simulink model "pathNavigation_PID_VEX"  (R2017a)
settings: Solver=FixedStepAuto  StartTime=0.0  StopTime=inf  FixedStep=Ts  RelTol=1e-3  EnableMultiTasking=on
PreLoadFcn:
  | robotParameters;
undefined symbols (not defined in the file or in its folder): axleLength, motorIp, motorSp, ticksPerRot, Ts, wheelR
libraries: vexarmcortexlib x8, simulink x2, simulink_extras x1, mobileRoboticsTrainingLib x1
settings Model: ExtModeTrigDuration=25  Creator=sseshadr  LastModifiedBy=shiremat
settings OptimizationCC: PassReuseOutputArgsAs=Individual arguments  MaxStackSize=64
settings DebuggingCC: ParameterTunabilityLossMsg=error
settings HardwareCC: ProdBitPerPointer=32  ProdBitPerSizeT=32  ProdBitPerPtrDiffT=32  ProdLargestAtomicInteger=Long  ProdLargestAtomicFloat=Double  ProdWordSize=32  ProdHWDeviceType=ARM Compatible->ARM Cortex
settings SFSimCC: MATLABDynamicMemAlloc=off
settings RTWCC: SystemTargetFile=ert.tlc  HardwareBoard=ARM Cortex-based VEX Microcontroller  TLCOptions="-aInlineSetEventsForThisBaseRateFcn=TLC_FALSE -aSuppressMultiTaskScheduler=TLC_FALSE  -aRateBasedStepFcn=0"  TemplateMakefile=ert_default_tmf  Description=Embedded Coder  GenerateReport=on  Toolchain=GNU Tools for VEX ARM Cortex  IncludeHyperlinkInReport=on  LaunchReport=on  GenerateTraceInfo=on  GenerateTraceReport=on  GenerateTraceReportSl=on  GenerateTraceReportSf=on  GenerateTraceReportEml=on
settings CodeAppCC: ForceParamTrailComments=on  IgnoreCustomStorageClasses=off  OperatorAnnotations=on  SimulinkDataObjDesc=on  SFDataObjDesc=on  MATLABFcnDesc=on  InsertBlockDesc=on  MATLABSourceComments=on

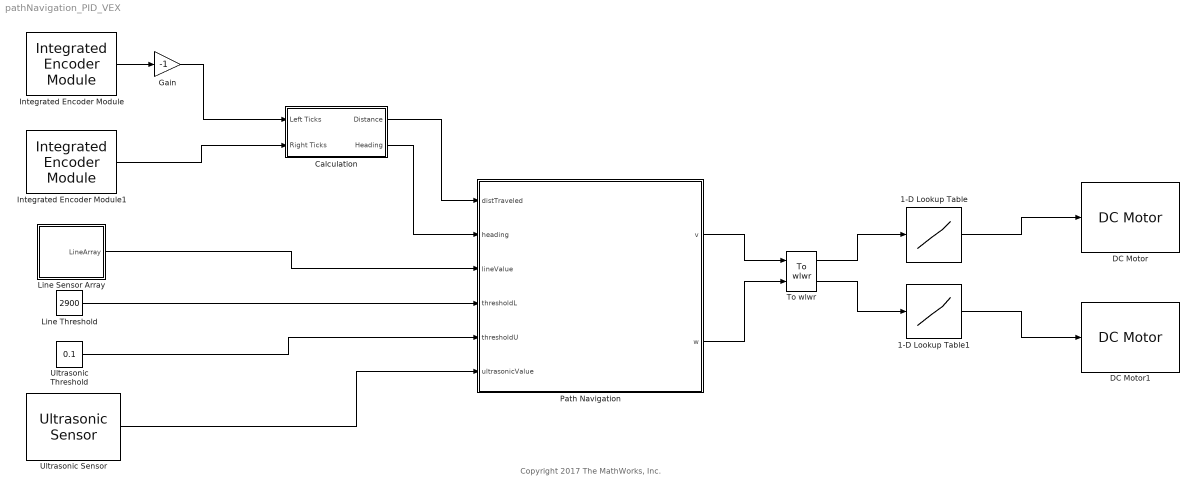
== system pathNavigation_PID_VEX ==
  note: Copyright 2017 The MathWorks, Inc.
  1-D Lookup Table : Lookup_n-D  NumberOfTableDimensions=1  BreakpointsForDimension1=motorSp  Table=motorIp  ExtrapMethod=Clip  InternalRulePriority=Speed  RndMeth=Simplest  InputSameDT=on
  1-D Lookup Table1 : Lookup_n-D  NumberOfTableDimensions=1  BreakpointsForDimension1=motorSp  Table=motorIp  ExtrapMethod=Clip  InternalRulePriority=Speed  RndMeth=Simplest  InputSameDT=on
  Calculation : Subsystem
  DC Motor : vexarmcortexlib/Actuators/DC Motor  motor=10  scaleFactor=1/13.5  SimulationOut=off
      settings: SourceProductName=Simulink Coder Support Package for ARM Cortex-based VEX Microcontroller  SourceProductBaseCode=EC_VEX_MICRO
  DC Motor1 : vexarmcortexlib/Actuators/DC Motor  motor=1  scaleFactor=1/13.5  SimulationOut=off
      settings: SourceProductName=Simulink Coder Support Package for ARM Cortex-based VEX Microcontroller  SourceProductBaseCode=EC_VEX_MICRO
  Gain : Gain  Gain=-1
  Integrated Encoder Module : vexarmcortexlib/Sensors/Integrated Encoder Module  motorType=VEX 393 (High torque)  seqNumI2C=1  resetOption=No reset  rotVelocity=off  inputPortSim=off  SampleTime=Ts
      settings: SourceProductName=Simulink Coder Support Package for ARM Cortex-based VEX Microcontroller  SourceProductBaseCode=EC_VEX_MICRO
  Integrated Encoder Module1 : vexarmcortexlib/Sensors/Integrated Encoder Module  motorType=VEX 393 (High torque)  seqNumI2C=0  resetOption=No reset  rotVelocity=off  inputPortSim=off  SampleTime=Ts
      settings: SourceProductName=Simulink Coder Support Package for ARM Cortex-based VEX Microcontroller  SourceProductBaseCode=EC_VEX_MICRO
  Line Sensor Array : Subsystem
  Line Threshold : Constant  Value=2900
  Path Navigation : Stateflow chart  TreatAsAtomicUnit=on
  To wlwr : mobileRoboticsTrainingLib/To wlwr  axleLength=axleLength  wheelR=wheelR
  Ultrasonic Sensor : vexarmcortexlib/Sensors/Ultrasonic Sensor  inputPin=7  outputPin=6  inputPortSim=off  SampleTime=Ts
      settings: SourceProductName=Simulink Coder Support Package for ARM Cortex-based VEX Microcontroller  SourceProductBaseCode=EC_VEX_MICRO
  Ultrasonic Threshold : Constant  Value=0.1
  wires:
  1-D Lookup Table1/1 -> DC Motor1/1
  1-D Lookup Table/1 -> DC Motor/1
  To wlwr/1 -> 1-D Lookup Table/1
  To wlwr/2 -> 1-D Lookup Table1/1
  Path Navigation/1(v) -> To wlwr/1
  Path Navigation/2(w) -> To wlwr/2
  Ultrasonic Sensor/1 -> Path Navigation/6(ultrasonicValue)
  Integrated Encoder Module1/1 -> Calculation/2(Right Ticks)
  Integrated Encoder Module/1 -> Gain/1
  Calculation/1(Distance) -> Path Navigation/1(distTraveled)
  Calculation/2(Heading) -> Path Navigation/2(heading)
  Line Threshold/1 -> Path Navigation/4(thresholdL)
  Ultrasonic Threshold/1 -> Path Navigation/5(thresholdU)
  Gain/1 -> Calculation/1(Left Ticks)
  Line Sensor Array/1(LineArray) -> Path Navigation/3(lineValue)

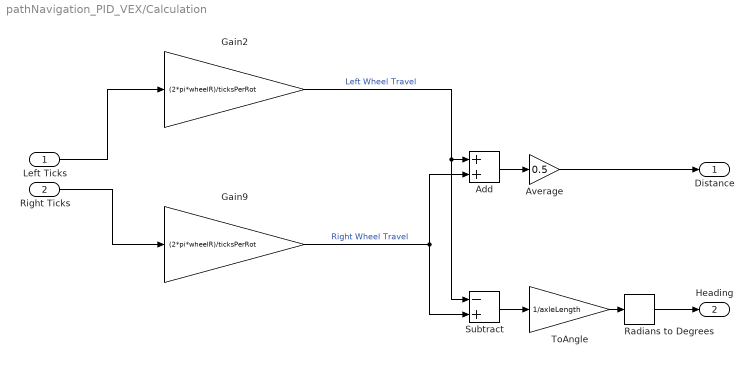
== system pathNavigation_PID_VEX/Calculation ==
  Left Ticks : Inport
  Right Ticks : Inport  Port=2
  Add : Sum
  Average : Gain  Gain=0.5
  Gain2 : Gain  Gain=(2*pi*wheelR)/ticksPerRot
  Gain9 : Gain  Gain=(2*pi*wheelR)/ticksPerRot
  Radians to Degrees : simulink_extras/Transformations/Radians to Degrees
  Subtract : Sum  Inputs=-+
  ToAngle : Gain  Gain=1/axleLength
  Distance : Outport
  Heading : Outport  Port=2
  wires:
  Average/1 -> Distance/1
  Add/1 -> Average/1
  Gain2/1 -> Subtract/1, Add/1  "Left Wheel Travel"
  Right Ticks/1 -> Gain9/1
  Left Ticks/1 -> Gain2/1
  Gain9/1 -> Subtract/2, Add/2  "Right Wheel Travel"
  Subtract/1 -> ToAngle/1
  ToAngle/1 -> Radians to Degrees/1
  Radians to Degrees/1 -> Heading/1

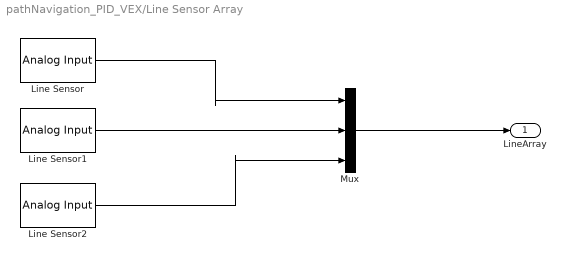
== system pathNavigation_PID_VEX/Line Sensor Array ==
  Line Sensor : vexarmcortexlib/Sensors/Analog Input  inChan=8  SimulationIn=off  SampleTime=Ts
      settings: SourceProductName=Simulink Coder Support Package for ARM Cortex-based VEX Microcontroller  SourceProductBaseCode=EC_VEX_MICRO
  Line Sensor1 : vexarmcortexlib/Sensors/Analog Input  inChan=7  SimulationIn=off  SampleTime=Ts
      settings: SourceProductName=Simulink Coder Support Package for ARM Cortex-based VEX Microcontroller  SourceProductBaseCode=EC_VEX_MICRO
  Line Sensor2 : vexarmcortexlib/Sensors/Analog Input  inChan=6  SimulationIn=off  SampleTime=Ts
      settings: SourceProductName=Simulink Coder Support Package for ARM Cortex-based VEX Microcontroller  SourceProductBaseCode=EC_VEX_MICRO
  Mux : Mux  Inputs=3
  LineArray : Outport
  wires:
  Line Sensor1/1 -> Mux/2
  Line Sensor/1 -> Mux/1
  Line Sensor2/1 -> Mux/3
  Mux/1 -> LineArray/1

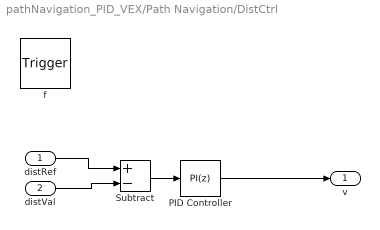
== system pathNavigation_PID_VEX/Path Navigation/DistCtrl ==
  distRef : Inport  OutDataTypeStr=double  PortDimensions=1
  distVal : Inport  Port=2  OutDataTypeStr=double  PortDimensions=1
  f : TriggerPort  TriggerType=function-call  VariantControl=Variant
      settings: CopyFcn=Stateflow.SLINSF.SimulinkMan.removeBlockPreDeleteFcn  PreDeleteFcn=Stateflow.SLINSF.SimulinkMan.unsafePredeleteFcn
  PID Controller : simulink/Continuous/PID Controller  Controller=PI  TimeDomain=Discrete-time  SampleTime=-1  IntegratorMethod=Forward Euler  FilterMethod=Forward Euler  Form=Parallel  UseFilter=off  ControllerParametersSource=internal  P=1.1  I=0.2  D=-0.0140783779685636  N=151.701833251505  InitialConditionSource=internal  InitialConditionForIntegrator=0  InitialConditionForFilter=0  ExternalReset=none  LimitOutput=on  UpperSaturationLimit=0.6  LowerSaturationLimit=-0.6  LinearizeAsGain=on  AntiWindupMode=clamping  Kb=1  TrackingMode=off  Kt=1  PParamMin=[]  PParamMax=[]  IParamMin=[]  IParamMax=[]  DParamMin=[]  DParamMax=[]  NParamMin=[]  NParamMax=[]  KbParamMin=[]  KbParamMax=[]  KtParamMin=[]  KtParamMax=[]  POutMin=[]  POutMax=[]  IOutMin=[]  IOutMax=[]  DOutMin=[]  DOutMax=[]  NOutMin=[]  NOutMax=[]  KbOutMin=[]  KbOutMax=[]  KtOutMin=[]  KtOutMax=[]  IntegratorOutMin=[]  IntegratorOutMax=[]  FilterOutMin=[]  FilterOutMax=[]  SumOutMin=[]  SumOutMax=[]  SumI1OutMin=[]  SumI1OutMax=[]  SumI2OutMin=[]  SumI2OutMax=[]  SumI3OutMin=[]  SumI3OutMax=[]  SumDOutMin=[]  SumDOutMax=[]  SaturationOutMin=[]  SaturationOutMax=[]  IntegratorContinuousStateAttributes=''  IntegratorStateMustResolveToSignalObject=off  IntegratorRTWStateStorageClass=Auto  FilterContinuousStateAttributes=''  FilterStateMustResolveToSignalObject=off  FilterRTWStateStorageClass=Auto  DifferentiatorICPrevScaledInput=0  DifferentiatorOutMin=[]  DifferentiatorOutMax=[]  InitialConditionSetting=Output
  Subtract : Sum  Inputs=+-
  v : Outport
  wires:
  Subtract/1 -> PID Controller/1
  PID Controller/1 -> v/1
  distRef/1 -> Subtract/1
  distVal/1 -> Subtract/2

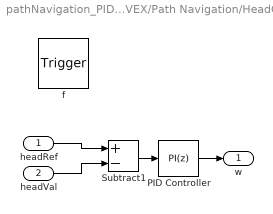
== system pathNavigation_PID_VEX/Path Navigation/HeadCtrl ==
  headRef : Inport  OutDataTypeStr=double  PortDimensions=1
  headVal : Inport  Port=2  OutDataTypeStr=double  PortDimensions=1
  f : TriggerPort  TriggerType=function-call  VariantControl=Variant
      settings: CopyFcn=Stateflow.SLINSF.SimulinkMan.removeBlockPreDeleteFcn  PreDeleteFcn=Stateflow.SLINSF.SimulinkMan.unsafePredeleteFcn
  PID Controller : simulink/Continuous/PID Controller  Controller=PI  TimeDomain=Discrete-time  SampleTime=-1  IntegratorMethod=Forward Euler  FilterMethod=Forward Euler  Form=Parallel  UseFilter=off  ControllerParametersSource=internal  P=0.1  I=0.1  D=-0.0140783779685636  N=151.701833251505  InitialConditionSource=internal  InitialConditionForIntegrator=0  InitialConditionForFilter=0  ExternalReset=none  LimitOutput=on  UpperSaturationLimit=4  LowerSaturationLimit=-4  LinearizeAsGain=on  AntiWindupMode=clamping  Kb=1  TrackingMode=off  Kt=1  PParamMin=[]  PParamMax=[]  IParamMin=[]  IParamMax=[]  DParamMin=[]  DParamMax=[]  NParamMin=[]  NParamMax=[]  KbParamMin=[]  KbParamMax=[]  KtParamMin=[]  KtParamMax=[]  POutMin=[]  POutMax=[]  IOutMin=[]  IOutMax=[]  DOutMin=[]  DOutMax=[]  NOutMin=[]  NOutMax=[]  KbOutMin=[]  KbOutMax=[]  KtOutMin=[]  KtOutMax=[]  IntegratorOutMin=[]  IntegratorOutMax=[]  FilterOutMin=[]  FilterOutMax=[]  SumOutMin=[]  SumOutMax=[]  SumI1OutMin=[]  SumI1OutMax=[]  SumI2OutMin=[]  SumI2OutMax=[]  SumI3OutMin=[]  SumI3OutMax=[]  SumDOutMin=[]  SumDOutMax=[]  SaturationOutMin=[]  SaturationOutMax=[]  IntegratorContinuousStateAttributes=''  IntegratorStateMustResolveToSignalObject=off  IntegratorRTWStateStorageClass=Auto  FilterContinuousStateAttributes=''  FilterStateMustResolveToSignalObject=off  FilterRTWStateStorageClass=Auto  DifferentiatorICPrevScaledInput=0  DifferentiatorOutMin=[]  DifferentiatorOutMax=[]  InitialConditionSetting=Output
  Subtract1 : Sum  Inputs=+-
  w : Outport
  wires:
  Subtract1/1 -> PID Controller/1
  PID Controller/1 -> w/1
  headRef/1 -> Subtract1/1
  headVal/1 -> Subtract1/2

== stateflow chart pathNavigation_PID_VEX/Path Navigation ==
  state SegmentA
    state MoveForward
      entry:
      v = DistCtrl(1.05,distTraveled);
    state Stop
      entry:
      v = 0;
    state Rotate
      entry:
      w = HeadCtrl(-85,heading);
    state Stop1
      entry:
      w = 0;
    (default) -> SegmentA.MoveForward : %Start Dead Reckoning
    SegmentA.MoveForward -> SegmentA.Stop : [distTraveled >= 1.05]
    SegmentA.Stop -> SegmentA.Rotate
    SegmentA.Rotate -> SegmentA.Stop1 : [heading <= -85]
  state v = DistCtrl(distRef,distVal) [function]
  state w = HeadCtrl(headRef,headVal) [function]
  state SegmentB
    state FindLine
      entry:
      v = 0.15;
    state GoLeft
      entry:
      v = 0.15;
      w = 1.5;
    state GoRight
      entry:
      v = 0.15;
      w = -1.5;
    state Stop
      entry:
      v = 0;
      w = 0;
    (default) -> FindLine
    FindLine -> GoLeft : [lineValue(2) > thresholdL]
    GoLeft -> GoRight [order 1] : [lineValue(2) < thresholdL]
    GoRight -> GoLeft [order 1] : [lineValue(2) >= thresholdL]
    GoLeft -> SegmentB.Stop [order 2] : [all(lineValue > thresholdL)]
    GoRight -> SegmentB.Stop [order 2] : [all(lineValue > thresholdL)]
  state SegmentC
    state MoveForward
      entry:
      v = 0.15;
      currDist = distTraveled;
    state Stop
      entry:
      v = 0;
    state Rotate
      entry:
      w = 1.5;
      currHead = heading;
    state Stop1
      entry:
      w = 0;
    (default) -> SegmentC.MoveForward : %Start Dead Reckoning
    SegmentC.MoveForward -> SegmentC.Stop : [distTraveled - currDist >= 0.4]
    SegmentC.Stop -> SegmentC.Rotate
    SegmentC.Rotate -> SegmentC.Stop1 : [heading - currHead >= 45]
  state SegmentD
    state Go
      entry: v = 0.2;
    state Stop
      entry: v = 0;
    (default) -> Go
    Go -> SegmentD.Stop : [ultrasonicValue <= thresholdU && ultrasonicValue > 0]
  (default) -> SegmentA
  SegmentA.Stop1 -> SegmentB
  SegmentB.Stop -> SegmentC
  SegmentC.Stop1 -> SegmentD
  data: distRef function_input double size=1; distVal function_input double size=1; v function_output; headRef function_input double size=1; headVal function_input double size=1; w function_output; distTraveled input; heading input; lineValue input; thresholdL input; thresholdU input; ultrasonicValue input; v output; w output; currDist local; currHead local
